simulink model "sim_traj_nonlin"  (R2025b)
settings: Solver=VariableStepAuto  StartTime=0.0  StopTime=10.0  RelTol=1e-3
undefined symbols (not defined in the file): Ts
settings Model: Creator=noyan  LastModifiedBy=noyan

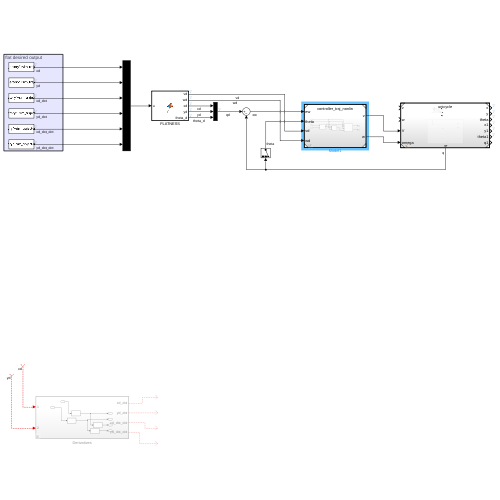
[thumbnail: Simulink's stored preview of the top-level diagram]
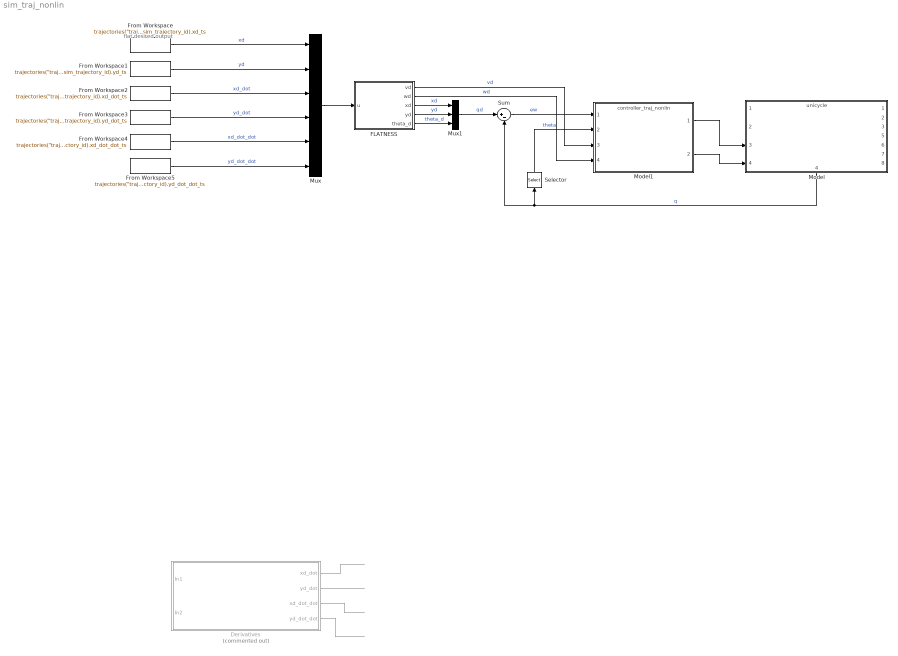
== system sim_traj_nonlin ==
  note: flat desired output
  Derivatives : Subsystem  Commented=on
  FLATNESS : MATLAB Function  TreatAsAtomicUnit=on
  From Workspace : FromWorkspace  VariableName="trajectories(\"trajectory\"+sim_trajectory_id).xd_ts"  SampleTime=Ts  OutputAfterFinalValue=Holding final value
  From Workspace1 : FromWorkspace  VariableName="trajectories(\"trajectory\"+sim_trajectory_id).yd_ts"  SampleTime=Ts  OutputAfterFinalValue=Holding final value
  From Workspace2 : FromWorkspace  VariableName="trajectories(\"trajectory\"+sim_trajectory_id).xd_dot_ts"  SampleTime=Ts  OutputAfterFinalValue=Holding final value
  From Workspace3 : FromWorkspace  VariableName="trajectories(\"trajectory\"+sim_trajectory_id).yd_dot_ts"  SampleTime=Ts  OutputAfterFinalValue=Holding final value
  From Workspace4 : FromWorkspace  VariableName="trajectories(\"trajectory\"+sim_trajectory_id).xd_dot_dot_ts"  SampleTime=Ts  OutputAfterFinalValue=Holding final value
  From Workspace5 : FromWorkspace  VariableName="trajectories(\"trajectory\"+sim_trajectory_id).yd_dot_dot_ts"  SampleTime=Ts  OutputAfterFinalValue=Holding final value
  Model : ModelReference  ModelNameDialog=unicycle.slx  SimulationMode=Normal  ModelReferenceVersion=1.11
      settings: PortSchema="{\"entries\":[{\"content\":{\"sides\":[{\"content\":{\"connectorIds\":[\"In1\",\"In2\",\"In3\",\"In4\"]},\"type\":\"ConnectorPlacement.EquallySpacedRectSide\",\"uuid\":\"ad25d81c-9301-4260-b0e7-6964e2a4144d\"},{\"content\":{\"connectorIds\":[\"Out1\",\"Out2\",\"Out3\",\"Out5\",\"Out6\",\"Out7\",\"Out8\"],\"side\":\"RIGHT\"},\"type\":\"ConnectorPlacement.EquallySpacedRectSide\",\"uuid\":\"e119e278-1a19-4d21-ac57-f30b4b2846c4\"},{\"content\":{\"side\":\"TOP\"},\"type\":\"ConnectorPlacement.EquallySpacedRectSide\",\"uuid\":\"f58ebd06-2844-4b35-9f44-2944c544d228\"},{\"content\":{\"connectorIds\":[\"Out4\"],\"side\":\"BOTTOM\"},\"type\":\"ConnectorPlacement.EquallySpacedRectSide\",\"uuid\":\"e9666c6b-2f60-424a-96df-bac3fd1a20e8\"}]},\"type\":\"ConnectorPlacement.EquallySpacedConnector\",\"uuid\":\"feeb8aec-4c5e-4f88-9f0a-836c4fc89b7c\"}],\"packageUris\":[\"http://schema.mathworks.com/mf0/Connector/R2020b\"],\"version\":\"1.0\"}"
  Model1 : ModelReference  ModelNameDialog=controller_traj_nonlin.slx  SimulationMode=Normal  ModelReferenceVersion=1.21
  Mux : Mux  Inputs=6
  Mux1 : Mux  Inputs=3
  Selector : Selector  InputPortWidth=3  IndexOptions=Index vector (dialog)  Indices=[3]  OutputSizes=1
  Sum : Sum  Inputs=|+-
  wires:
  FLATNESS/5(theta_d) -> Mux1/3  "theta_d"
  FLATNESS/4(yd) -> Mux1/2  "yd"
  From Workspace1/1 -> Mux/2  "yd"
  FLATNESS/3(xd) -> Mux1/1  "xd"
  From Workspace/1 -> Mux/1  "xd"
  Sum/1 -> Model1/1  "ew"
  Selector/1 -> Model1/2  "theta"
  FLATNESS/2(wd) -> Model1/4  "wd"
  Mux/1 -> FLATNESS/1(u)
  Mux1/1 -> Sum/1  "qd"
  FLATNESS/1(vd) -> Model1/3  "vd"
  Derivatives/1(xd_dot) -> ?
  ? -> Derivatives/2(In2)  "yd"
  ? -> Derivatives/1(In1)  "xd"
  Derivatives/4(yd_dot_dot) -> ?
  Derivatives/2(yd_dot) -> ?
  Derivatives/3(xd_dot_dot) -> ?
  From Workspace2/1 -> Mux/3  "xd_dot"
  From Workspace3/1 -> Mux/4  "yd_dot"
  From Workspace4/1 -> Mux/5  "xd_dot_dot"
  From Workspace5/1 -> Mux/6  "yd_dot_dot"
  Model1/1 -> Model/3
  Model1/2 -> Model/4
  Model/4 -> Selector/1, Sum/2  "q"

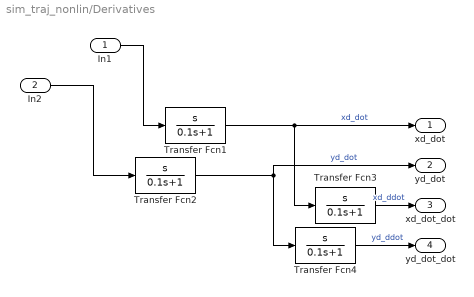
== system sim_traj_nonlin/Derivatives ==
  In1 : Inport
  In2 : Inport  Port=2
  Transfer Fcn{1..4} (4 alike) : TransferFcn  Numerator=[1 0]  Denominator=[0.1 1]
  xd_dot : Outport
  yd_dot : Outport  Port=2
  xd_dot_dot : Outport  Port=3
  yd_dot_dot : Outport  Port=4
  wires:
  Transfer Fcn3/1 -> xd_dot_dot/1  "xd_ddot"
  Transfer Fcn1/1 -> xd_dot/1, Transfer Fcn3/1  "xd_dot"
  Transfer Fcn2/1 -> yd_dot/1, Transfer Fcn4/1  "yd_dot"
  Transfer Fcn4/1 -> yd_dot_dot/1  "yd_ddot"
  In1/1 -> Transfer Fcn1/1
  In2/1 -> Transfer Fcn2/1

== matlab function sim_traj_nonlin/FLATNESS ==
  data: u input; vd output; wd output; xd output; yd output; theta_d output
function [vd, wd, xd, yd, theta_d]= fcn(u)

xd_dot = u(3);
yd_dot= u(4);
xd_dot_dot = u(5);
yd_dot_dot= u(6);

v = sqrt(xd_dot^2 + yd_dot^2);
w = (xd_dot*yd_dot_dot - xd_dot_dot*yd_dot) / max(xd_dot^2 + yd_dot^2, 1e-3);



vd = v;
wd = w;
xd = u(1);
yd = u(2);
theta_d = atan2(yd_dot, xd_dot);
